simulink model "Quadcopter"  (R2025a)
settings: Solver=ode23t  StartTime=0.0  StopTime=15  RelTol=1e-2  EnableMultiTasking=on
values from neighbouring files (symbols this model uses):
  IC = struct    [IC_custom_setup.m]
  Tf = 10    [QuadParametersRL.m]    (also in Train_DDPG.m = 15; uavScenario_simulation.m = 120)
  Ts = 0.005    [QuadParametersRL.m]    (also in Train_DDPG.m; uavScenario_simulation.m)
undefined symbols (not defined in the file or in its folder): quadModel
libraries: simulink x15, rllib x1
settings Model: SimulationMode=accelerator  Creator=The MathWorks, Inc.  LastModifiedBy=yachiashen
settings SolverCC: ZeroCrossAlgorithm=Adaptive  AlgebraicLoopSolver=TrustRegion
settings DataIOCC: SaveOutput=off  SignalLogging=off  DSMLogging=off  SaveTime=off  ReturnWorkspaceOutputs=off  OutputTimes=0:0.01:10
settings OptimizationCC: LifeSpan=inf
settings DebuggingCC: MaxConsecutiveZCsMsg=warning  IgnoredZcDiagnostic=none  UnconnectedInputMsg=warning  UnconnectedOutputMsg=warning  UnconnectedLineMsg=warning  AllowSymbolicDim=off  SFUnexpectedBacktrackingDiag=warning  SFNoUnconditionalDefaultTransitionDiag=warning  SFExecutionAtInitializationDiag=none  UnitsInconsistencyMsg=none  ArithmeticOperatorsInVariantConditions=warning
settings ModelReferenceCC: EnableRefExpFcnMdlSchedulingChecks=on
settings SFSimCC: SimUseLocalCustomCode=off  CustomCodeUndefinedFunction=UseInterfaceOnly
settings RTWCC: RTWUseLocalCustomCode=off  GPUComputeCapability=3.5
settings CodeAppCC: StateflowObjectComments=on
settings GRTTargetCC: TargetLangStandard=C89/C90 (ANSI)
settings ConfigComp: CovMetricSettings=dw  CovSaveCumulativeToWorkspaceVar=on  CovSaveSingleToWorkspaceVar=on  CovExternalEMLEnable=off  CovSFcnEnable=off
settings SimscapeCC: SimscapeNormalizeSystem=off  SimscapeLogOpenViewer=on  SimscapeLogLimitData=off  SimscapeLogDataHistory=10000.0
settings ConfigurationSet: Description=SimMechanics 2G
settings DiagnosticsConfigSet: SimMechanicsRigidlyBoundBlock=none
settings ExplorerConfigSet: SimMechanicsOpenEditorOnUpdate=off  InternalSimMechanicsExplorerSettings="<ExplorerConfiguration><canonicalview>default</canonicalview><AnimationSetting><BasePlaybackSpeed>1.0</BasePlaybackSpeed><PlaybackSpeedFactor>1.0</PlaybackSpeedFactor></AnimationSetting><TilePanel><TileInfo><Tiles Columns=\"1\" Count=\"1\" Rows=\"1\"><Column Weight=\"1\"/><Row Weight=\"1\"/><Tile Height=\"1\" Width=\"1\" X=\"0\" Y=\"0\"/></Tiles></TileInfo><SceneInfo><SceneViewer><BGColor><R>0.60000002384185791</R><G>0.60000002384185791</G><B>0.60000002384185791</B></BGColor><Camera><DoPerspective>off</DoPerspective><Position><X>7.18002534815406079</X><Y>-8.21011991112170847</Y><Z>8.33180938462712462</Z></Position><Center><X>1.10741005252516134</X><Y>-0.176829942633513204</Y><Z>0.646464709811595872</Z></Center><Up><X>-0.335329266167064488</X><Y>0.506481739462631531</Y><Z>0.79437430147428989</Z></Up><ViewLimDist>1</ViewLimDist><YLim>0.739205014828661411</YLim><XLim>1.12849377732657596</XLim></Camera></SceneViewer></SceneInfo></TilePanel><MechEditorPanel><Cameras/><GfxPanelCameraMap/><VideoCreator><PlaybackSpeedRatio>1.0</PlaybackSpeedRatio><FrameRate>30</FrameRate><VideoFormat>Motion JPEG AVI</VideoFormat><FrameSize>auto</FrameSize></VideoCreator></MechEditorPanel></ExplorerConfiguration>"

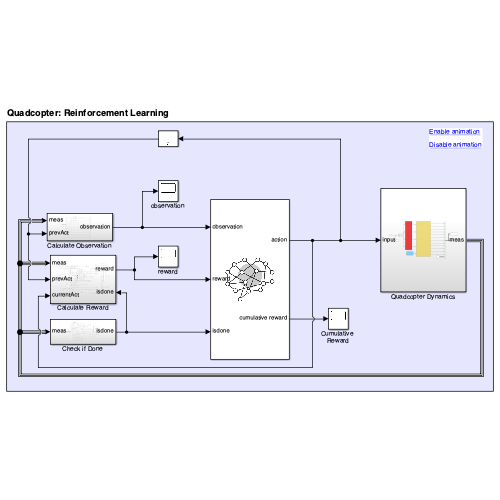
[thumbnail: Simulink's stored preview of the top-level diagram]
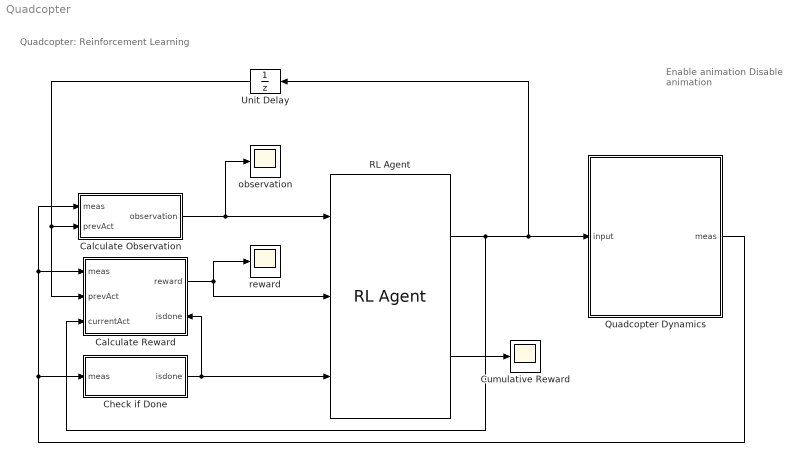
== system Quadcopter ==
  note: Enable animation
      |
      | Disable animation
  note: Quadcopter: Reinforcement Learning
  Calculate Observation : Subsystem
  Calculate Reward : Subsystem
      settings: PortSchema="{\"entries\":[{\"content\":{\"sides\":[{\"content\":{\"connectorIds\":[\"In1\",\"In2\",\"In3\"]},\"type\":\"ConnectorPlacement.EquallySpacedRectSide\",\"uuid\":\"eba832e6-c0a7-4400-bc7d-e99d6fe1f5c9\"},{\"content\":{\"connectorIds\":[\"Out1\",\"In4\"],\"side\":\"RIGHT\"},\"type\":\"ConnectorPlacement.EquallySpacedRectSide\",\"uuid\":\"28aa866f-cf6c-43de-96f5-ac1b7cc26ea1\"},{\"content\":{\"side\":\"TOP\"},\"type\":\"ConnectorPlacement.EquallySpacedRectSide\",\"uuid\":\"ec249893-a602-489f-835a-2a652f38a2b1\"}]},\"type\":\"ConnectorPlacement.EquallySpacedConnector\",\"uuid\":\"b2df43a5-a7e7-4182-9e82-9901ef84ccaa\"}],\"packageUris\":[\"http://schema.mathworks.com/mf0/Connector/R2020b\"],\"version\":\"1.0\"}"
  Check if Done : Subsystem
  Cumulative Reward : Scope
      settings: ActiveDisplayYMinimum=-1368.76702  ActiveDisplayYMaximum=152.08522
  Quadcopter Dynamics : Subsystem
  RL Agent : rllib/RL Agent  Agent=agent  ExternalActionAsInput=off  ProvideLastAction=off  ProvideCumRwd=on  TreatAsDirectFeedthrough=on  UseStrictObservationDataTypes=off
  Unit Delay : UnitDelay  SampleTime=-1  HasFrameUpgradeWarning=on
  observation : Scope
      settings: ActiveDisplayYMinimum=-8.81223  ActiveDisplayYMaximum=4.3658
  reward : Scope
      settings: ActiveDisplayYMinimum=-103.49713  ActiveDisplayYMaximum=11.49968  DataLoggingVariableName=ScopeData2
  wires:
  Calculate Reward/1(reward) -> RL Agent/2, reward/1
  Calculate Observation/1(observation) -> observation/1, RL Agent/1
  Check if Done/1(isdone) -> Calculate Reward/4(isdone), RL Agent/3
  RL Agent/2 -> Cumulative Reward/1
  Unit Delay/1 -> Calculate Observation/2(prevAct), Calculate Reward/2(prevAct)
  Quadcopter Dynamics/1(meas) -> Calculate Observation/1(meas), Calculate Reward/1(meas), Check if Done/1(meas)
  RL Agent/1 -> Calculate Reward/3(currentAct), Unit Delay/1, Quadcopter Dynamics/1(input)

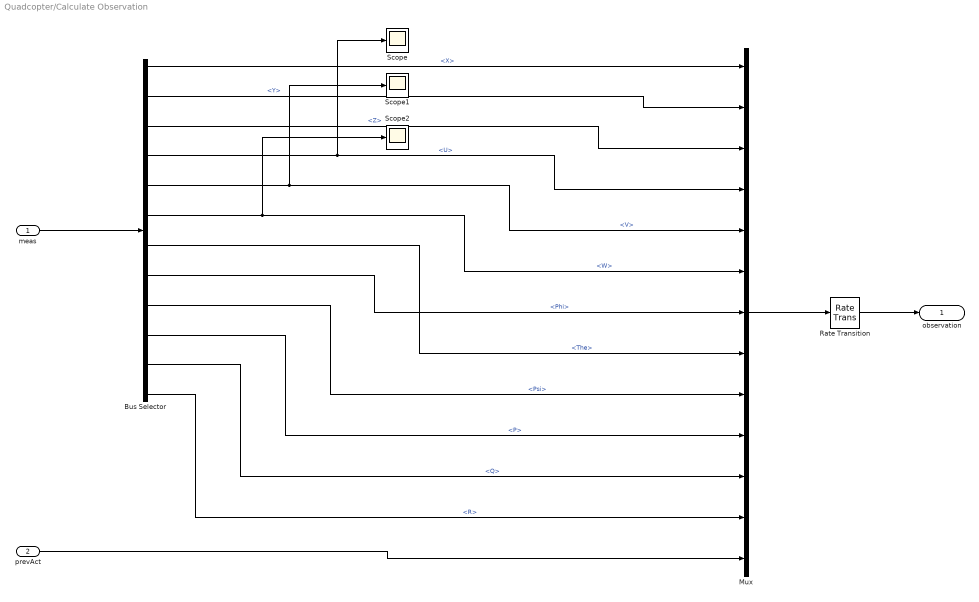
== system Quadcopter/Calculate Observation ==
  meas : Inport
  prevAct : Inport  Port=2
  Bus Selector : BusSelector  OutputSignals=X,Y,Z,U,V,W,The,Phi,Psi,P,Q,R
  Mux : Mux  Inputs=13
  Rate Transition : RateTransition
  Scope : Scope
      settings: ActiveDisplayYMinimum=-3.10574  ActiveDisplayYMaximum=1.94473  DataLoggingVariableName=ScopeData8
  Scope1 : Scope
      settings: ActiveDisplayYMinimum=-4.37438  ActiveDisplayYMaximum=5.00653  DataLoggingVariableName=ScopeData9
  Scope2 : Scope
      settings: ActiveDisplayYMinimum=-5.01889  ActiveDisplayYMaximum=4.98406  DataLoggingVariableName=ScopeData10
  observation : Outport  VectorParamsAs1DForOutWhenUnconnected=off
  wires:
  meas/1 -> Bus Selector/1
  Mux/1 -> Rate Transition/1
  Rate Transition/1 -> observation/1
  prevAct/1 -> Mux/13
  Bus Selector/3 -> Mux/3  "<Z>"
  Bus Selector/11 -> Mux/11  "<Q>"
  Bus Selector/12 -> Mux/12  "<R>"
  Bus Selector/1 -> Mux/1  "<X>"
  Bus Selector/4 -> Scope/1, Mux/4  "<U>"
  Bus Selector/2 -> Mux/2  "<Y>"
  Bus Selector/5 -> Scope1/1, Mux/5  "<V>"
  Bus Selector/6 -> Scope2/1, Mux/6  "<W>"
  Bus Selector/7 -> Mux/8  "<The>"
  Bus Selector/8 -> Mux/7  "<Phi>"
  Bus Selector/9 -> Mux/9  "<Psi>"
  Bus Selector/10 -> Mux/10  "<P>"

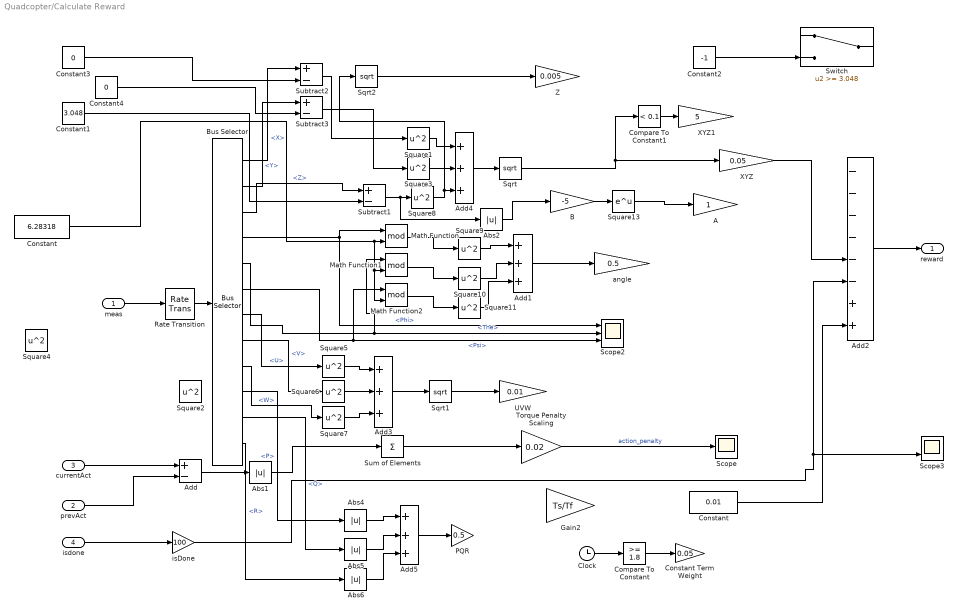
== system Quadcopter/Calculate Reward ==
  meas : Inport
  prevAct : Inport  Port=2
  currentAct : Inport  Port=3
  isdone : Inport  Port=4
  A : Gain
  Abs{1..2,4..6} (5 alike) : Abs  SaturateOnIntegerOverflow=off
  Add : Sum  Inputs=+-
  Add{1,3..5} (4 alike) : Sum  Inputs=+++
  Add2 : Sum  Inputs=------++
  B : Gain  Gain=-5
  Bus Selector : BusSelector  OutputSignals=X,Y,Z,Phi,The,Psi,U,V,W,P,Q,R
  Clock : Clock
  Compare To Constant : simulink/Logic and Bit Operations/Compare To Constant  relop=>=  const=1.8  OutDataTypeStr=boolean
  Compare To Constant1 : simulink/Logic and Bit Operations/Compare To Constant  relop=<  const=0.1  OutDataTypeStr=boolean
  Constant : Constant  Value=6.28318
  "Constant " : Constant  Value=0.01  SampleTime=-1
  Constant Term Weight : Gain  Gain=0.05
  Constant1 : Constant  Value=3.048
  Constant2 : Constant  Value=-1
  Constant3 : Constant  Value=0
  Constant4 : Constant  Value=0
  Gain2 : Gain  Gain=Ts/Tf
  Math Function : Math  Operator=mod
  Math Function1 : Math  Operator=mod
  Math Function2 : Math  Operator=mod
  PQR : Gain  Gain=0.5
  Rate Transition : RateTransition  OutPortSampleTime=Ts
  Scope : Scope
      settings: ActiveDisplayYMinimum=-0.52642  ActiveDisplayYMaximum=4.77282  DataLoggingVariableName=ScopeData2
  Scope2 : Scope  NumInputPorts=3
      settings: ActiveDisplayYMinimum=-13.191246815710164  ActiveDisplayYMaximum=2.3753600417367986  DataLoggingVariableName=ScopeData4
  Scope3 : Scope  NumInputPorts=2
      settings: ActiveDisplayYMinimum=-1  ActiveDisplayYMaximum=1  DataLoggingVariableName=ScopeData11
  Sqrt : Sqrt
  Sqrt1 : Sqrt
  Sqrt2 : Sqrt
  Square{1..11} (11 alike) : Math  Operator=square  SignedPower=on
  Square13 : Math  SignedPower=on
  Subtract1 : Sum  Inputs=+-
  Subtract2 : Sum  Inputs=+-
  Subtract3 : Sum  Inputs=+-
  Sum of Elements : Sum  Inputs=+
  Switch : Switch  Threshold=3.048  SaturateOnIntegerOverflow=off  InputSameDT=off
  Torque Penalty Scaling : Gain  Gain=0.02
  UVW : Gain  Gain=0.01
  XYZ : Gain  Gain=0.05
  XYZ1 : Gain  Gain=5
  Z : Gain  Gain=0.005
  angle : Gain  Gain=0.5
  isDone : Gain  Gain=100
  reward : Outport  VectorParamsAs1DForOutWhenUnconnected=off
  wires:
  meas/1 -> Rate Transition/1
  Rate Transition/1 -> Bus Selector/1
  Add2/1 -> reward/1
  Sum of Elements/1 -> Torque Penalty Scaling/1
  Bus Selector/3 -> Subtract1/1  "<Z>"
  Constant1/1 -> Subtract1/2
  Square1/1 -> Add4/1
  Square3/1 -> Add4/2
  Bus Selector/4 -> Math Function/1, Scope2/1  "<Phi>"
  Bus Selector/5 -> Math Function1/1, Scope2/2  "<The>"
  Bus Selector/6 -> Scope2/3, Math Function2/1  "<Psi>"
  Add1/1 -> angle/1
  Torque Penalty Scaling/1 -> Scope/1  "action_penalty"
  Constant2/1 -> Switch/3
  prevAct/1 -> Add/2
  currentAct/1 -> Add/1
  Add/1 -> Abs1/1
  Abs1/1 -> Sum of Elements/1
  isdone/1 -> isDone/1
  Subtract1/1 -> Abs2/1, Square8/1
  Square8/1 -> Add4/3, Sqrt2/1
  Add4/1 -> Sqrt/1
  Sqrt/1 -> Compare To Constant1/1, XYZ/1
  Square10/1 -> Add1/2
  Square9/1 -> Add1/1
  Bus Selector/7 -> Square5/1  "<U>"
  Bus Selector/8 -> Square6/1  "<V>"
  Bus Selector/9 -> Square7/1  "<W>"
  Square6/1 -> Add3/2
  Square5/1 -> Add3/1
  Square7/1 -> Add3/3
  Add3/1 -> Sqrt1/1
  Sqrt1/1 -> UVW/1
  Abs4/1 -> Add5/1
  Abs5/1 -> Add5/2
  Abs6/1 -> Add5/3
  Add5/1 -> PQR/1
  Bus Selector/10 -> Abs4/1  "<P>"
  Bus Selector/11 -> Abs5/1  "<Q>"
  Bus Selector/12 -> Abs6/1  "<R>"
  Clock/1 -> Compare To Constant/1
  Compare To Constant/1 -> Constant Term Weight/1
  Square11/1 -> Add1/3
  isDone/1 -> Scope3/2, Add2/6
  Constant/1 -> Math Function1/2, Math Function2/2, Math Function/2
  Math Function/1 -> Square9/1
  Math Function1/1 -> Square10/1
  Math Function2/1 -> Square11/1
  Sqrt2/1 -> Z/1
  B/1 -> Square13/1
  Square13/1 -> A/1
  Abs2/1 -> B/1
  Subtract2/1 -> Square1/1
  Bus Selector/1 -> Subtract2/1  "<X>"
  Bus Selector/2 -> Subtract3/1  "<Y>"
  Subtract3/1 -> Square3/1
  Compare To Constant1/1 -> XYZ1/1
  Constant3/1 -> Subtract2/2
  Constant4/1 -> Subtract3/2
  "Constant "/1 -> Add2/8
  XYZ/1 -> Add2/5

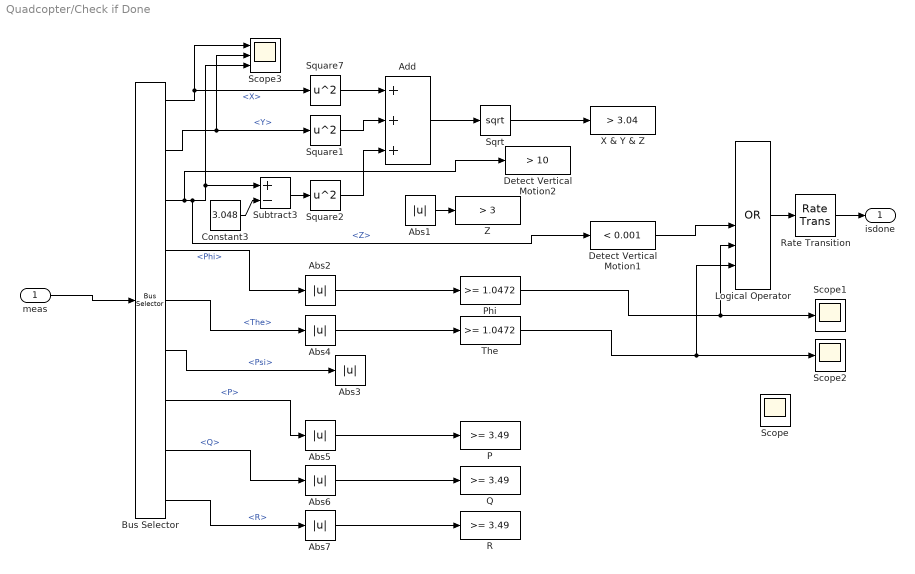
== system Quadcopter/Check if Done ==
  meas : Inport
  Abs{1..7} (7 alike) : Abs  SaturateOnIntegerOverflow=off
  Add : Sum  Inputs=+++
  Bus Selector : BusSelector  OutputSignals=X,Y,Z,Phi,The,Psi,P,Q,R
  Constant3 : Constant  Value=3.048
  Detect Vertical Motion1 : simulink/Logic and Bit Operations/Compare To Constant  relop=<  const=0.001  OutDataTypeStr=boolean
  Detect Vertical Motion2 : simulink/Logic and Bit Operations/Compare To Constant  relop=>  const=10  OutDataTypeStr=boolean
  Logical Operator : Logic  Operator=OR  Inputs=8  AllPortsSameDT=off  OutDataTypeStr=boolean
  P : simulink/Logic and Bit Operations/Compare To Constant  relop=>=  const=3.49  OutDataTypeStr=boolean
  Phi : simulink/Logic and Bit Operations/Compare To Constant  relop=>=  const=1.0472  OutDataTypeStr=boolean
  Q : simulink/Logic and Bit Operations/Compare To Constant  relop=>=  const=3.49  OutDataTypeStr=boolean
  R : simulink/Logic and Bit Operations/Compare To Constant  relop=>=  const=3.49  OutDataTypeStr=boolean
  Rate Transition : RateTransition
  Scope : Scope
      settings: ActiveDisplayYMinimum=-1  ActiveDisplayYMaximum=1
  Scope1 : Scope
      settings: ActiveDisplayYMinimum=-1  ActiveDisplayYMaximum=1  DataLoggingVariableName=ScopeData2
  Scope2 : Scope
      settings: ActiveDisplayYMinimum=-1  ActiveDisplayYMaximum=1  DataLoggingVariableName=ScopeData3
  Scope3 : Scope  NumInputPorts=3
      settings: ActiveDisplayYMinimum=-0.38099999999999989  ActiveDisplayYMaximum=3.4290000000000003  DataLoggingVariableName=ScopeData12
  Sqrt : Sqrt
  Square1 : Math  Operator=square  SignedPower=on
  Square2 : Math  Operator=square  SignedPower=on
  Square7 : Math  Operator=square  SignedPower=on
  Subtract3 : Sum  Inputs=+-
  The : simulink/Logic and Bit Operations/Compare To Constant  relop=>=  const=1.0472  OutDataTypeStr=boolean
  X & Y & Z : simulink/Logic and Bit Operations/Compare To Constant  relop=>  const=3.04  OutDataTypeStr=boolean
  Z : simulink/Logic and Bit Operations/Compare To Constant  relop=>  const=3  OutDataTypeStr=boolean
  isdone : Outport  VectorParamsAs1DForOutWhenUnconnected=off
  wires:
  meas/1 -> Bus Selector/1
  Rate Transition/1 -> isdone/1
  Bus Selector/1 -> Scope3/1, Square7/1  "<X>"
  Bus Selector/2 -> Scope3/2, Square1/1  "<Y>"
  Abs2/1 -> Phi/1
  Bus Selector/4 -> Abs2/1  "<Phi>"
  Abs4/1 -> The/1
  Bus Selector/5 -> Abs4/1  "<The>"
  The/1 -> Scope2/1, Logical Operator/7
  Constant3/1 -> Subtract3/2
  Abs1/1 -> Z/1
  Square7/1 -> Add/1
  Square1/1 -> Add/2
  Add/1 -> Sqrt/1
  Sqrt/1 -> X & Y & Z/1
  Logical Operator/1 -> Rate Transition/1
  Bus Selector/7 -> Abs5/1  "<P>"
  Bus Selector/3 -> Detect Vertical Motion2/1, Detect Vertical Motion1/1, Scope3/3, Subtract3/1  "<Z>"
  Abs5/1 -> P/1
  Abs6/1 -> Q/1
  Abs7/1 -> R/1
  Bus Selector/9 -> Abs7/1  "<R>"
  Bus Selector/8 -> Abs6/1  "<Q>"
  Bus Selector/6 -> Abs3/1  "<Psi>"
  Subtract3/1 -> Square2/1
  Square2/1 -> Add/3
  Phi/1 -> Logical Operator/6, Scope1/1
  Detect Vertical Motion1/1 -> Logical Operator/5

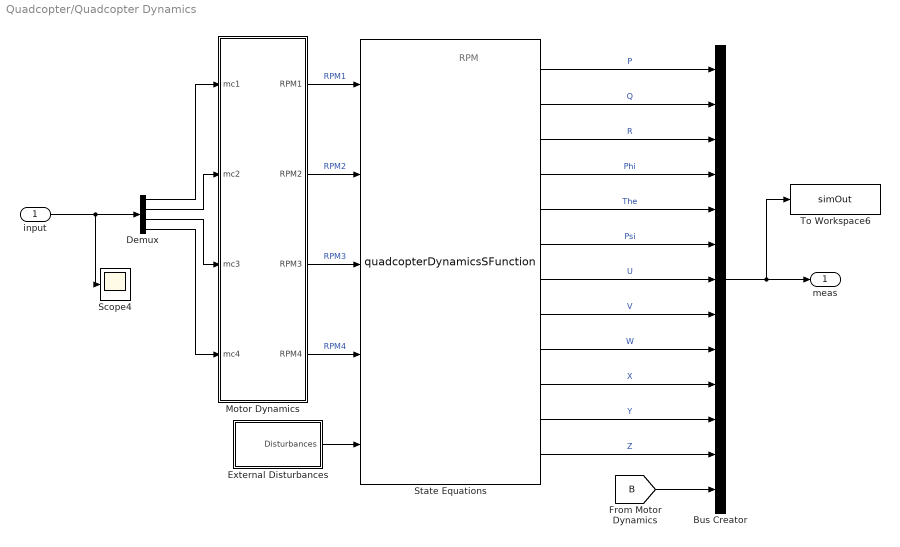
== system Quadcopter/Quadcopter Dynamics ==
  note: RPM
  input : Inport
  Bus Creator : BusCreator  Inputs=13
  Demux : Demux
  External Disturbances : Subsystem
  Motor Dynamics : Subsystem
  Scope4 : Scope
      settings: ActiveDisplayYMinimum=-12.48463  ActiveDisplayYMaximum=112.49829
  State Equations : M-S-Function  FunctionName=quadcopterDynamicsSFunction  Parameters=quadModel, IC
      mask Display:
      | port_label('input', 1, 'RPM1')
      | port_label('input', 2, 'RPM2')
      | port_label('input', 3, 'RPM3')
      | port_label('input', 4, 'RPM4')
      | port_label('input', 5, 'Disturbances')
      | port_label('output', 1, 'P')
      | port_label('output', 2, 'Q')
      | port_label('output', 3, 'R')
      | port_label('output', 4, 'Phi')
      | port_label('output', 5, 'The')
      | port_label('output', 6, 'Psi')
      | port_label('output', 7, 'U')
      | port_label('output', 8, 'V')
      | port_label('output', 9, 'W')
      | port_label('output', 10, 'X')
      | port_label('output', 11, 'Y')
      | port_label('output', 12, 'Z')
  To Workspace6 : ToWorkspace  VariableName=simOut  SaveFormat=Structure With Time  SampleTime=-1
      settings: Save2DSignal=2-D array (concatenate along first dimension)
  meas : Outport
  wires:
  Bus Creator/1 -> meas/1, To Workspace6/1
  External Disturbances/1("Disturbances ") -> State Equations/5
  Motor Dynamics/1(RPM1) -> State Equations/1  "RPM1"
  Motor Dynamics/3(RPM3) -> State Equations/3  "RPM3"
  Motor Dynamics/2(RPM2) -> State Equations/2  "RPM2"
  State Equations/10 -> Bus Creator/10  "X"
  [B] -> Bus Creator/13
  State Equations/12 -> Bus Creator/12  "Z"
  State Equations/7 -> Bus Creator/7  "U"
  State Equations/3 -> Bus Creator/3  "R"
  State Equations/8 -> Bus Creator/8  "V"
  State Equations/1 -> Bus Creator/1  "P"
  State Equations/9 -> Bus Creator/9  "W"
  State Equations/11 -> Bus Creator/11  "Y"
  State Equations/5 -> Bus Creator/5  "The"
  State Equations/6 -> Bus Creator/6  "Psi"
  State Equations/2 -> Bus Creator/2  "Q"
  State Equations/4 -> Bus Creator/4  "Phi"
  Motor Dynamics/4(RPM4) -> State Equations/4  "RPM4"
  Demux/1 -> Motor Dynamics/1(mc1)
  Demux/2 -> Motor Dynamics/2(mc2)
  input/1 -> Scope4/1, Demux/1
  Demux/3 -> Motor Dynamics/3(mc3)
  Demux/4 -> Motor Dynamics/4(mc4)

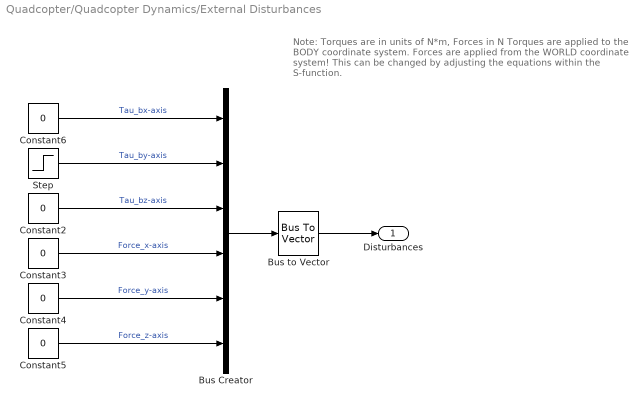
== system Quadcopter/Quadcopter Dynamics/External Disturbances ==
  note: Note: Torques are in units of N*m, Forces in N
      | Torques are applied to the BODY coordinate system.
      | Forces are applied from the WORLD coordinate system!
      | This can be changed by adjusting the equations within the S-function.
  Bus Creator : BusCreator  Inputs=6
  Bus to Vector : BusToVector
  Constant{2..6} (5 alike) : Constant  Value=0
  Step : Step  After=0  SampleTime=0
  "Disturbances " : Outport
  wires:
  Constant5/1 -> Bus Creator/6  "Force_z-axis"
  Constant4/1 -> Bus Creator/5  "Force_y-axis"
  Constant3/1 -> Bus Creator/4  "Force_x-axis"
  Constant2/1 -> Bus Creator/3  "Tau_bz-axis"
  Step/1 -> Bus Creator/2  "Tau_by-axis"
  Constant6/1 -> Bus Creator/1  "Tau_bx-axis"
  Bus Creator/1 -> Bus to Vector/1
  Bus to Vector/1 -> "Disturbances "/1

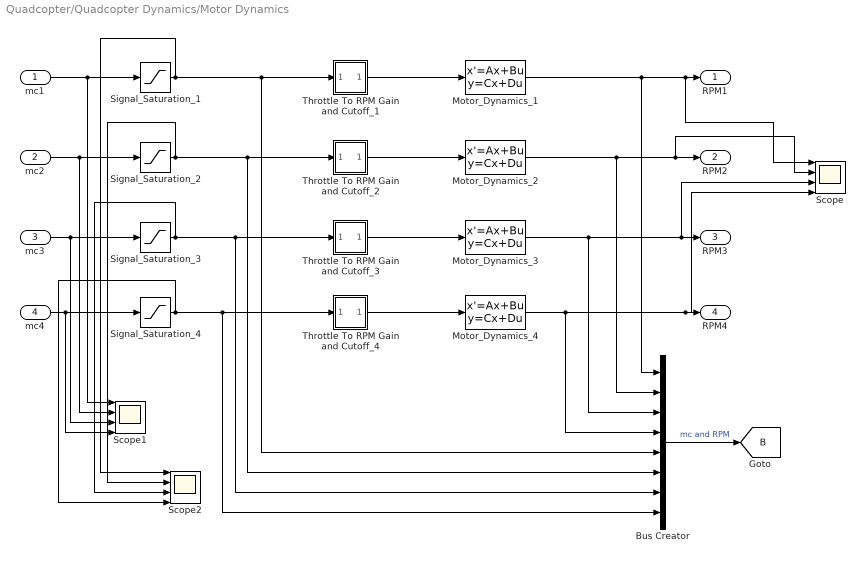
== system Quadcopter/Quadcopter Dynamics/Motor Dynamics ==
  mc1 : Inport
  mc2 : Inport  Port=2
  mc3 : Inport  Port=3
  mc4 : Inport  Port=4
  Bus Creator : BusCreator  Inputs=8
  Motor_Dynamics_1 : StateSpace  A=-1/quadModel.T  C=1/quadModel.T  D=0  InitialCondition=IC.w1*quadModel.T
  Motor_Dynamics_2 : StateSpace  A=-1/quadModel.T  C=1/quadModel.T  D=0  InitialCondition=IC.w2*quadModel.T
  Motor_Dynamics_3 : StateSpace  A=-1/quadModel.T  C=1/quadModel.T  D=0  InitialCondition=IC.w3*quadModel.T
  Motor_Dynamics_4 : StateSpace  A=-1/quadModel.T  C=1/quadModel.T  D=0  InitialCondition=IC.w4*quadModel.T
  Scope : Scope  NumInputPorts=4
      settings: ActiveDisplayYMinimum=2411.365  ActiveDisplayYMaximum=4176.515  DataLoggingVariableName=ScopeData5
  Scope1 : Scope  NumInputPorts=4
      settings: ActiveDisplayYMinimum=-12.5  ActiveDisplayYMaximum=112.5  DataLoggingVariableName=ScopeData6
  Scope2 : Scope  NumInputPorts=4
      settings: ActiveDisplayYMinimum=-12.5  ActiveDisplayYMaximum=112.5  DataLoggingVariableName=ScopeData7
  Signal_Saturation_{1..4} (4 alike) : Saturate  UpperLimit=100  LowerLimit=0
  Throttle To RPM Gain and Cutoff_1 : Subsystem
  Throttle To RPM Gain and Cutoff_2 : Subsystem
  Throttle To RPM Gain and Cutoff_3 : Subsystem
  Throttle To RPM Gain and Cutoff_4 : Subsystem
  RPM1 : Outport
  RPM2 : Outport  Port=2
  RPM3 : Outport  Port=3
  RPM4 : Outport  Port=4
  tag scope: B=global
  wires:
  Bus Creator/1 -> [B]  "mc and RPM"
  Motor_Dynamics_4/1 -> Scope/4, RPM4/1, Bus Creator/4
  Motor_Dynamics_3/1 -> Scope/3, RPM3/1, Bus Creator/3
  Motor_Dynamics_2/1 -> Scope/2, RPM2/1, Bus Creator/2
  Motor_Dynamics_1/1 -> Scope/1, RPM1/1, Bus Creator/1
  Throttle To RPM Gain and Cutoff_4/1(Out5) -> Motor_Dynamics_4/1
  Throttle To RPM Gain and Cutoff_3/1(Out5) -> Motor_Dynamics_3/1
  Throttle To RPM Gain and Cutoff_2/1(Out5) -> Motor_Dynamics_2/1
  Signal_Saturation_4/1 -> Scope2/4, Throttle To RPM Gain and Cutoff_4/1(In5), Bus Creator/8
  Signal_Saturation_3/1 -> Scope2/3, Throttle To RPM Gain and Cutoff_3/1(In5), Bus Creator/7
  Signal_Saturation_2/1 -> Scope2/2, Throttle To RPM Gain and Cutoff_2/1(In5), Bus Creator/6
  Signal_Saturation_1/1 -> Scope2/1, Throttle To RPM Gain and Cutoff_1/1(In5), Bus Creator/5
  mc3/1 -> Scope1/3, Signal_Saturation_3/1
  mc2/1 -> Scope1/2, Signal_Saturation_2/1
  mc4/1 -> Scope1/4, Signal_Saturation_4/1
  mc1/1 -> Scope1/1, Signal_Saturation_1/1
  Throttle To RPM Gain and Cutoff_1/1(Out5) -> Motor_Dynamics_1/1

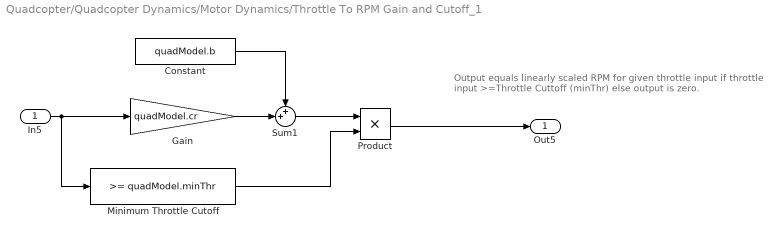
== system Quadcopter/Quadcopter Dynamics/Motor Dynamics/Throttle To RPM Gain and Cutoff_1 ==
  note: Output equals linearly scaled RPM
      | for given throttle input if throttle input >=Throttle Cuttoff (minThr)
      | else output is zero.
  In5 : Inport
  Constant : Constant  Value=quadModel.b
  Gain : Gain  Gain=quadModel.cr
  Minimum Throttle Cutoff : simulink/Logic and Bit Operations/Compare To Constant  relop=>=  const=quadModel.minThr  OutDataTypeStr=uint8
  Product : Product
  Sum1 : Sum  Inputs=++|
  Out5 : Outport
  wires:
  Constant/1 -> Sum1/1
  Sum1/1 -> Product/1
  Gain/1 -> Sum1/2
  In5/1 -> Minimum Throttle Cutoff/1, Gain/1
  Product/1 -> Out5/1
  Minimum Throttle Cutoff/1 -> Product/2

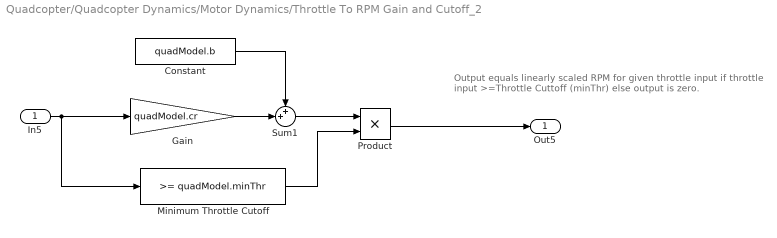
== system Quadcopter/Quadcopter Dynamics/Motor Dynamics/Throttle To RPM Gain and Cutoff_2 ==
  note: Output equals linearly scaled RPM
      | for given throttle input if throttle input >=Throttle Cuttoff (minThr)
      | else output is zero.
  In5 : Inport
  Constant : Constant  Value=quadModel.b
  Gain : Gain  Gain=quadModel.cr
  Minimum Throttle Cutoff : simulink/Logic and Bit Operations/Compare To Constant  relop=>=  const=quadModel.minThr  OutDataTypeStr=uint8
  Product : Product
  Sum1 : Sum  Inputs=++|
  Out5 : Outport
  wires:
  Constant/1 -> Sum1/1
  Sum1/1 -> Product/1
  Gain/1 -> Sum1/2
  In5/1 -> Minimum Throttle Cutoff/1, Gain/1
  Product/1 -> Out5/1
  Minimum Throttle Cutoff/1 -> Product/2

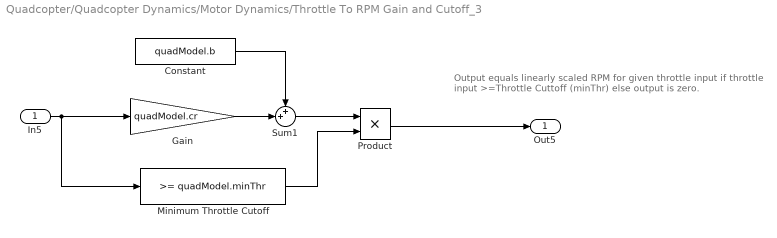
== system Quadcopter/Quadcopter Dynamics/Motor Dynamics/Throttle To RPM Gain and Cutoff_3 ==
  note: Output equals linearly scaled RPM
      | for given throttle input if throttle input >=Throttle Cuttoff (minThr)
      | else output is zero.
  In5 : Inport
  Constant : Constant  Value=quadModel.b
  Gain : Gain  Gain=quadModel.cr
  Minimum Throttle Cutoff : simulink/Logic and Bit Operations/Compare To Constant  relop=>=  const=quadModel.minThr  OutDataTypeStr=uint8
  Product : Product
  Sum1 : Sum  Inputs=++|
  Out5 : Outport
  wires:
  Constant/1 -> Sum1/1
  Sum1/1 -> Product/1
  Gain/1 -> Sum1/2
  In5/1 -> Minimum Throttle Cutoff/1, Gain/1
  Product/1 -> Out5/1
  Minimum Throttle Cutoff/1 -> Product/2

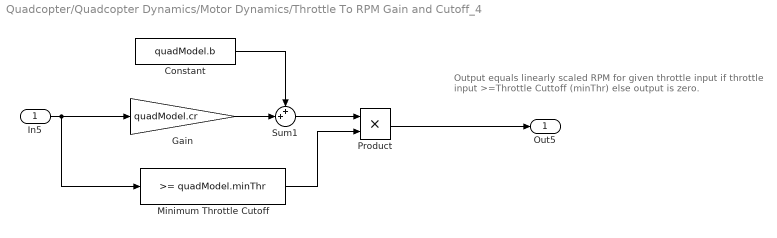
== system Quadcopter/Quadcopter Dynamics/Motor Dynamics/Throttle To RPM Gain and Cutoff_4 ==
  note: Output equals linearly scaled RPM
      | for given throttle input if throttle input >=Throttle Cuttoff (minThr)
      | else output is zero.
  In5 : Inport
  Constant : Constant  Value=quadModel.b
  Gain : Gain  Gain=quadModel.cr
  Minimum Throttle Cutoff : simulink/Logic and Bit Operations/Compare To Constant  relop=>=  const=quadModel.minThr  OutDataTypeStr=uint8
  Product : Product
  Sum1 : Sum  Inputs=++|
  Out5 : Outport
  wires:
  Constant/1 -> Sum1/1
  Sum1/1 -> Product/1
  Gain/1 -> Sum1/2
  In5/1 -> Minimum Throttle Cutoff/1, Gain/1
  Product/1 -> Out5/1
  Minimum Throttle Cutoff/1 -> Product/2
